simulink model "Modelo_LTI_Aumentado"  (R2021a)
settings: Solver=VariableStepAuto  StartTime=0.0  StopTime=10.0  RelTol=1e-3
undefined symbols (not defined in the file): beq, Cts, Jeq, lambda_m, Ld, Lq, Pp, r, Rs_40, Rts_amb
settings Model: Creator=fhlla  LastModifiedBy=fhlla

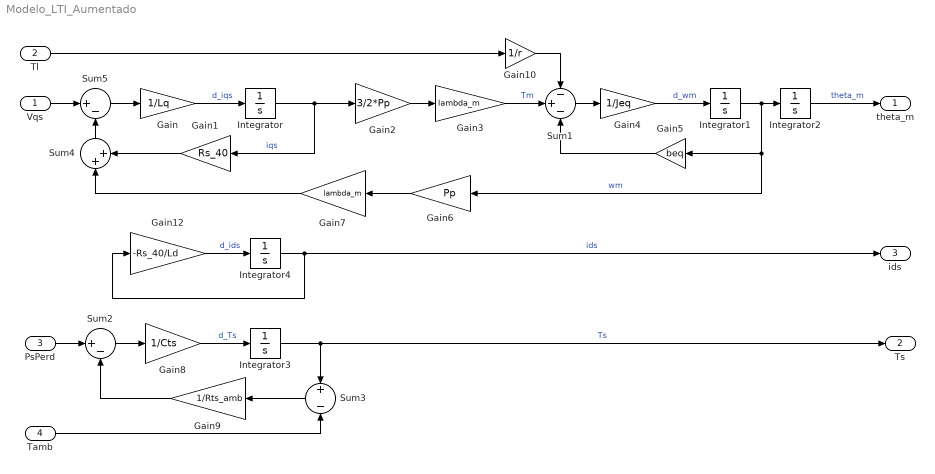
== system Modelo_LTI_Aumentado ==
  Vqs : Inport
  Tl : Inport  Port=2
  PsPerd : Inport  Port=3
  Tamb : Inport  Port=4
  Gain : Gain  Gain=1/Lq
  Gain1 : Gain  Gain=Rs_40
  Gain10 : Gain  Gain=1/r
  Gain12 : Gain  Gain=-Rs_40/Ld
  Gain2 : Gain  Gain=3/2*Pp
  Gain3 : Gain  Gain=lambda_m
  Gain4 : Gain  Gain=1/Jeq
  Gain5 : Gain  Gain=beq
  Gain6 : Gain  Gain=Pp
  Gain7 : Gain  Gain=lambda_m
  Gain8 : Gain  Gain=1/Cts
  Gain9 : Gain  Gain=1/Rts_amb
  Integrator{,1..4} (5 alike) : Integrator
  Sum1 : Sum  Inputs=-+-
  Sum2 : Sum  Inputs=|+-
  Sum3 : Sum  Inputs=+-
  Sum4 : Sum  Inputs=|++
  Sum5 : Sum  Inputs=|+-
  theta_m : Outport
  Ts : Outport  Port=2
  ids : Outport  Port=3
  wires:
  Sum5/1 -> Gain/1
  Gain/1 -> Integrator/1  "d_iqs"
  Gain2/1 -> Gain3/1
  Gain9/1 -> Sum2/2
  Gain1/1 -> Sum4/2
  Integrator1/1 -> Integrator2/1, Gain6/1, Gain5/1  "wm"
  Integrator/1 -> Gain1/1, Gain2/1  "iqs"
  Gain8/1 -> Integrator3/1  "d_Ts"
  Sum2/1 -> Gain8/1
  Gain3/1 -> Sum1/2  "Tm"
  Tl/1 -> Gain10/1
  Vqs/1 -> Sum5/1
  Sum3/1 -> Gain9/1
  Gain4/1 -> Integrator1/1  "d_wm"
  Tamb/1 -> Sum3/2
  Gain6/1 -> Gain7/1
  Sum1/1 -> Gain4/1
  Gain7/1 -> Sum4/1
  Integrator2/1 -> theta_m/1  "theta_m"
  PsPerd/1 -> Sum2/1
  Gain5/1 -> Sum1/3
  Sum4/1 -> Sum5/2
  Gain10/1 -> Sum1/1
  Integrator3/1 -> Ts/1, Sum3/1  "Ts"
  Gain12/1 -> Integrator4/1  "d_ids"
  Integrator4/1 -> ids/1, Gain12/1  "ids"
